simulink library "beamform"  (Simulink 7.0)
libraries: xbsIndex_r4 x65, beamform x13
settings Model: Creator=mdexter  LastModifiedBy=mdexter

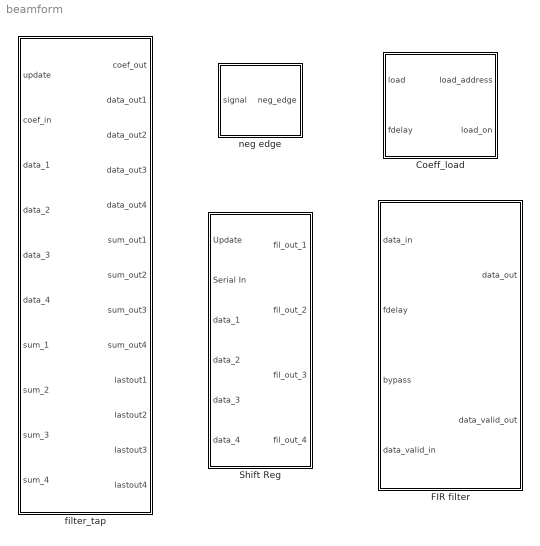
== system beamform ==
  Coeff_load : Subsystem  mask{nfilters=10, ntaps=20}
      mask prompts: nfilters "Number of FD filters"; ntaps "Number of Taps per filter"
      mask init:
      | coef_load;
  FIR filter : Subsystem
  Shift Reg : Subsystem  mask{n=10, bin_point=6}
      mask prompts: n "No of taps"; bin_point "Binary Point"
      mask init:
      | shift_reg;
  filter_tap : Subsystem  mask{n_bits=8, bnpnt=6, mux_latency=0, add_latency=2, mult_latency=3, qn_bits=18, qbnpnt=16}
      mask prompts: n_bits "Coefficient bit width"; bnpnt "Coeff & Data Binary Point"; mux_latency "Multiplexer Latency"; add_latency "Add Latency"; mult_latency "Multiplier Latency"; qn_bits "Quiscent Bitwdith"; qbnpnt "Quiscent Binary Point"
  neg edge : Subsystem  mask{add_latency=1}

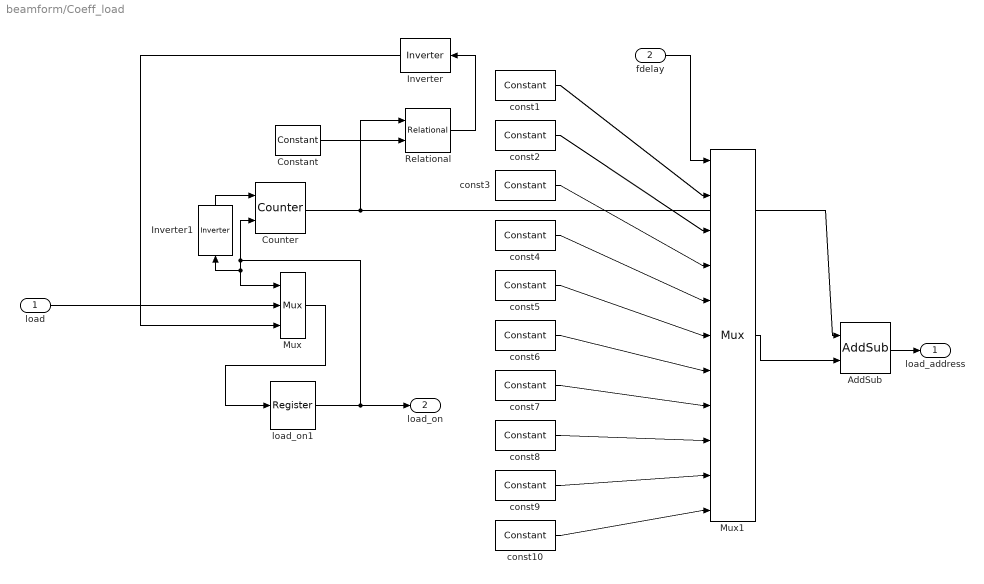
== system beamform/Coeff_load ==
  load : Inport  OutDataType=sfix(16)  OutScaling=2^0
  fdelay : Inport  Port=2  OutDataType=sfix(16)  OutScaling=2^0
  AddSub : xbsIndex_r4/AddSub  mode=Addition  use_carryin=off  use_carryout=off  en=off  latency=1  precision=User Defined  arith_type=Unsigned  n_bits=8  bin_pt=0  quantization=Truncate  overflow=Wrap  dbl_ovrd=off  use_behavioral_HDL=on  pipelined=off  use_rpm=on  hw_selection=Fabric  block_type=addsub
      settings: xl_area=[0, 0, 0, 0, 0, 0, 0]  block_version=10.1.3
  Constant : xbsIndex_r4/Constant  arith_type=Unsigned  const=19  n_bits=5  bin_pt=0  explicit_period=on  period=1  equ=P=C  opselect=C  inp2=PCIN>>17  opr=+  inp1=P  carry=CIN  dbl_ovrd=off  block_type=constant
  Counter : xbsIndex_r4/Counter  cnt_type=Count Limited  cnt_to=19  operation=Up  start_count=0  cnt_by_val=1  arith_type=Unsigned  n_bits=5  bin_pt=0  load_pin=off  rst=on  en=on  explicit_period=off  period=1  dbl_ovrd=off  use_behavioral_HDL=off  use_rpm=on  implementation=Fabric  block_type=counter
      settings: xl_area=[0, 0, 0, 0, 0, 0, 0]
  Inverter : xbsIndex_r4/Inverter  Orientation=left  en=off  latency=0  dbl_ovrd=off  block_type=inv
      settings: xl_area=[0, 0, 0, 0, 0, 0, 0]
  Inverter1 : xbsIndex_r4/Inverter  Orientation=up  en=off  latency=0  dbl_ovrd=off  block_type=inv
      settings: xl_area=[0, 0, 0, 0, 0, 0, 0]
  Mux : xbsIndex_r4/Mux  inputs=2  en=off  latency=0  precision=Full  arith_type="Signed  (2's comp)"  n_bits=8  bin_pt=2  quantization=Truncate  overflow=Wrap  dbl_ovrd=off  block_type=mux
      settings: xl_area=[0, 0, 0, 0, 0, 0, 0]
  Mux1 : xbsIndex_r4/Mux  inputs=10  en=off  latency=1  precision=Full  arith_type="Signed  (2's comp)"  n_bits=8  bin_pt=2  quantization=Truncate  overflow=Wrap  dbl_ovrd=off  block_type=mux
      settings: xl_area=[0, 0, 0, 0, 0, 0, 0]
  Relational : xbsIndex_r4/Relational  mode=a>=b  en=off  latency=1  dbl_ovrd=off  block_type=relational
      settings: xl_area=[0, 0, 0, 0, 0, 0, 0]  block_version=10.1.3
  const1 : xbsIndex_r4/Constant  arith_type=Unsigned  const=0  n_bits=8  bin_pt=0  explicit_period=off  period=1  equ=P=C  opselect=C  inp2=PCIN>>17  opr=+  inp1=P  carry=CIN  dbl_ovrd=off  block_type=constant
  const10 : xbsIndex_r4/Constant  arith_type=Unsigned  const=180  n_bits=8  bin_pt=0  explicit_period=off  period=1  equ=P=C  opselect=C  inp2=PCIN>>17  opr=+  inp1=P  carry=CIN  dbl_ovrd=off  block_type=constant
  const2 : xbsIndex_r4/Constant  arith_type=Unsigned  const=20  n_bits=8  bin_pt=0  explicit_period=off  period=1  equ=P=C  opselect=C  inp2=PCIN>>17  opr=+  inp1=P  carry=CIN  dbl_ovrd=off  block_type=constant
  const3 : xbsIndex_r4/Constant  arith_type=Unsigned  const=40  n_bits=8  bin_pt=0  explicit_period=off  period=1  equ=P=C  opselect=C  inp2=PCIN>>17  opr=+  inp1=P  carry=CIN  dbl_ovrd=off  block_type=constant
  const4 : xbsIndex_r4/Constant  arith_type=Unsigned  const=60  n_bits=8  bin_pt=0  explicit_period=off  period=1  equ=P=C  opselect=C  inp2=PCIN>>17  opr=+  inp1=P  carry=CIN  dbl_ovrd=off  block_type=constant
  const5 : xbsIndex_r4/Constant  arith_type=Unsigned  const=80  n_bits=8  bin_pt=0  explicit_period=off  period=1  equ=P=C  opselect=C  inp2=PCIN>>17  opr=+  inp1=P  carry=CIN  dbl_ovrd=off  block_type=constant
  const6 : xbsIndex_r4/Constant  arith_type=Unsigned  const=100  n_bits=8  bin_pt=0  explicit_period=off  period=1  equ=P=C  opselect=C  inp2=PCIN>>17  opr=+  inp1=P  carry=CIN  dbl_ovrd=off  block_type=constant
  const7 : xbsIndex_r4/Constant  arith_type=Unsigned  const=120  n_bits=8  bin_pt=0  explicit_period=off  period=1  equ=P=C  opselect=C  inp2=PCIN>>17  opr=+  inp1=P  carry=CIN  dbl_ovrd=off  block_type=constant
  const8 : xbsIndex_r4/Constant  arith_type=Unsigned  const=140  n_bits=8  bin_pt=0  explicit_period=off  period=1  equ=P=C  opselect=C  inp2=PCIN>>17  opr=+  inp1=P  carry=CIN  dbl_ovrd=off  block_type=constant
  const9 : xbsIndex_r4/Constant  arith_type=Unsigned  const=160  n_bits=8  bin_pt=0  explicit_period=off  period=1  equ=P=C  opselect=C  inp2=PCIN>>17  opr=+  inp1=P  carry=CIN  dbl_ovrd=off  block_type=constant
  load_on1 : xbsIndex_r4/Register  init=0  rst=off  en=off  dbl_ovrd=off  block_type=register
      settings: xl_area=[0, 0, 0, 0, 0, 0, 0]
  load_address : Outport  OutDataType=sfix(16)  OutScaling=2^0
  load_on : Outport  Port=2  OutDataType=sfix(16)  OutScaling=2^0
  wires:
  const10/1 -> Mux1/11
  const9/1 -> Mux1/10
  const8/1 -> Mux1/9
  const7/1 -> Mux1/8
  const6/1 -> Mux1/7
  const5/1 -> Mux1/6
  const4/1 -> Mux1/5
  const3/1 -> Mux1/4
  const2/1 -> Mux1/3
  const1/1 -> Mux1/2
  AddSub/1 -> load_address/1
  Mux1/1 -> AddSub/2
  fdelay/1 -> Mux1/1
  Inverter1/1 -> Counter/1
  load/1 -> Mux/2
  Mux/1 -> load_on1/1
  Inverter/1 -> Mux/3
  load_on1/1 -> load_on/1, Inverter1/1, Mux/1, Counter/2
  Relational/1 -> Inverter/1
  Constant/1 -> Relational/2
  Counter/1 -> AddSub/1, Relational/1

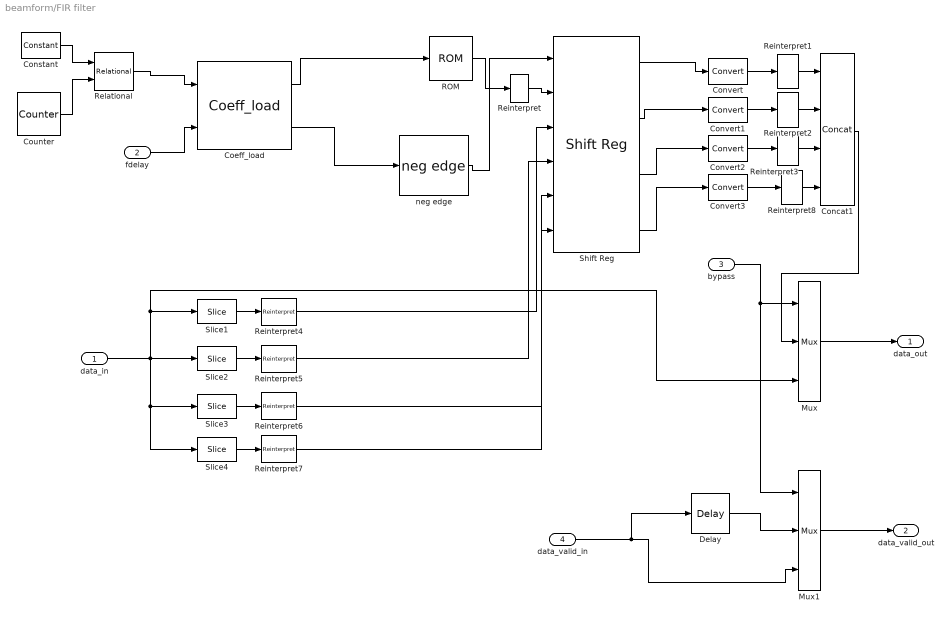
== system beamform/FIR filter ==
  data_in : Inport  OutDataType=sfix(16)  OutScaling=2^0
  fdelay : Inport  Port=2  OutDataType=sfix(16)  OutScaling=2^0
  bypass : Inport  Port=3  OutDataType=sfix(16)  OutScaling=2^0
  data_valid_in : Inport  Port=4  OutDataType=sfix(16)  OutScaling=2^0
  Coeff_load : beamform/Coeff_load  SystemSampleTime=-1  nfilters=10  ntaps=10
  Concat1 : xbsIndex_r4/Concat  num_inputs=4  dbl_ovrd=off  block_type=concat
      settings: block_version=10.1.3
  Constant : xbsIndex_r4/Constant  arith_type=Unsigned  const=0  n_bits=11  bin_pt=0  explicit_period=on  period=1  equ=P=C  opselect=C  inp2=PCIN>>17  opr=+  inp1=P  carry=CIN  dbl_ovrd=off  block_type=constant
  Convert{,1..3} (4 alike) : xbsIndex_r4/Convert  arith_type="Signed  (2's comp)"  n_bits=8  bin_pt=6  quantization=Truncate  overflow=Wrap  latency=0  dbl_ovrd=off  pipeline=off  block_type=convert
      settings: xl_area=[0, 0, 0, 0, 0, 0, 0]  block_version=10.1.3
  Counter : xbsIndex_r4/Counter  cnt_type=Free Running  cnt_to=Inf  operation=Up  start_count=0  cnt_by_val=1  arith_type=Unsigned  n_bits=11  bin_pt=0  load_pin=off  rst=off  en=off  explicit_period=off  period=1  dbl_ovrd=off  use_behavioral_HDL=off  use_rpm=on  implementation=Fabric  block_type=counter
      settings: xl_area=[0, 0, 0, 0, 0, 0, 0]
  Delay : xbsIndex_r4/Delay  en=off  latency=10*6  dbl_ovrd=off  reg_retiming=off  block_type=delay
      settings: xl_area=[0, 0, 0, 0, 0, 0, 0]
  Mux : xbsIndex_r4/Mux  inputs=2  en=off  latency=1  precision=Full  arith_type="Signed  (2's comp)"  n_bits=8  bin_pt=2  quantization=Truncate  overflow=Wrap  dbl_ovrd=off  block_type=mux
      settings: xl_area=[0, 0, 0, 0, 0, 0, 0]
  Mux1 : xbsIndex_r4/Mux  inputs=2  en=off  latency=1  precision=Full  arith_type="Signed  (2's comp)"  n_bits=8  bin_pt=2  quantization=Truncate  overflow=Wrap  dbl_ovrd=off  block_type=mux
      settings: xl_area=[0, 0, 0, 0, 0, 0, 0]
  ROM : xbsIndex_r4/ROM  depth=100  initVector=A  distributed_mem=Block RAM  rst=off  init_reg=0  en=off  latency=1  arith_type="Signed  (2's comp)"  n_bits=18  bin_pt=16  dbl_ovrd=off  optimize=Area  use_rpm=off  block_type=sprom
      settings: xl_area=[0, 0, 0, 0, 0, 0, 0]  block_version=10.1.3
  Reinterpret : xbsIndex_r4/Reinterpret  force_arith_type=on  arith_type="Signed  (2's comp)"  force_bin_pt=on  bin_pt=16  block_type=reinterpret
      settings: infoedit="Changes signal type without altering the binary representation.   You can changed the signal between signed and unsigned, and relocate the binary point.<P><P>Hardware notes: In hardware this block costs nothing.<P><P>Example:  Suppose the input is 6 bits wide, signed, with 2 fractional bits, and the output is forced to unsigned with 0 fractional bits.  Then an input of -2.0 (1110.00 in binary 2's complement) becomes an output of 56 (111000 in binary)."  block_version=10.1.3
  Reinterpret{1..3,8} (4 alike) : xbsIndex_r4/Reinterpret  force_arith_type=on  arith_type=Unsigned  force_bin_pt=on  bin_pt=0  block_type=reinterpret
      settings: infoedit="Changes signal type without altering the binary representation.   You can changed the signal between signed and unsigned, and relocate the binary point.<P><P>Hardware notes: In hardware this block costs nothing.<P><P>Example:  Suppose the input is 6 bits wide, signed, with 2 fractional bits, and the output is forced to unsigned with 0 fractional bits.  Then an input of -2.0 (1110.00 in binary 2's complement) becomes an output of 56 (111000 in binary)."  block_version=10.1.3
  Reinterpret{4..7} (4 alike) : xbsIndex_r4/Reinterpret  force_arith_type=on  arith_type="Signed  (2's comp)"  force_bin_pt=on  bin_pt=6  block_type=reinterpret
      settings: infoedit="Changes signal type without altering the binary representation.   You can changed the signal between signed and unsigned, and relocate the binary point.<P><P>Hardware notes: In hardware this block costs nothing.<P><P>Example:  Suppose the input is 6 bits wide, signed, with 2 fractional bits, and the output is forced to unsigned with 0 fractional bits.  Then an input of -2.0 (1110.00 in binary 2's complement) becomes an output of 56 (111000 in binary)."  block_version=10.1.3
  Relational : xbsIndex_r4/Relational  mode=a=b  en=off  latency=1  dbl_ovrd=off  block_type=relational
      settings: xl_area=[0, 0, 0, 0, 0, 0, 0]  block_version=10.1.3
  Shift Reg : beamform/Shift Reg  SystemSampleTime=-1  n=10  bin_point=6
  Slice1 : xbsIndex_r4/Slice  nbits=8  boolean_output=off  mode=Two Bit Locations  bit1=31  base1=LSB of Input  bit0=24  base0=LSB of Input  dbl_ovrd=off  block_type=slice
      settings: infoedit="Extracts a given range of bits from each input sample and presents it at the output.  The output type is ordinarily unsigned with binary point at zero, but can be Boolean when the slice is one bit wide.<P><P>Hardware notes: In hardware this block costs nothing."  block_version=10.1.3
  Slice2 : xbsIndex_r4/Slice  nbits=8  boolean_output=off  mode=Two Bit Locations  bit1=23  base1=LSB of Input  bit0=16  base0=LSB of Input  dbl_ovrd=off  block_type=slice
      settings: infoedit="Extracts a given range of bits from each input sample and presents it at the output.  The output type is ordinarily unsigned with binary point at zero, but can be Boolean when the slice is one bit wide.<P><P>Hardware notes: In hardware this block costs nothing."  block_version=10.1.3
  Slice3 : xbsIndex_r4/Slice  nbits=8  boolean_output=off  mode=Two Bit Locations  bit1=15  base1=LSB of Input  bit0=8  base0=LSB of Input  dbl_ovrd=off  block_type=slice
      settings: infoedit="Extracts a given range of bits from each input sample and presents it at the output.  The output type is ordinarily unsigned with binary point at zero, but can be Boolean when the slice is one bit wide.<P><P>Hardware notes: In hardware this block costs nothing."  block_version=10.1.3
  Slice4 : xbsIndex_r4/Slice  nbits=8  boolean_output=off  mode=Two Bit Locations  bit1=7  base1=LSB of Input  bit0=0  base0=LSB of Input  dbl_ovrd=off  block_type=slice
      settings: infoedit="Extracts a given range of bits from each input sample and presents it at the output.  The output type is ordinarily unsigned with binary point at zero, but can be Boolean when the slice is one bit wide.<P><P>Hardware notes: In hardware this block costs nothing."  block_version=10.1.3
  neg edge : beamform/neg edge  SystemSampleTime=-1  add_latency=1
  data_out : Outport  OutDataType=sfix(16)  OutScaling=2^0
  data_valid_out : Outport  Port=2  OutDataType=sfix(16)  OutScaling=2^0
  wires:
  Reinterpret/1 -> Shift Reg/2
  neg edge/1 -> Shift Reg/1
  Relational/1 -> Coeff_load/1
  Coeff_load/1 -> ROM/1
  ROM/1 -> Reinterpret/1
  Coeff_load/2 -> neg edge/1
  fdelay/1 -> Coeff_load/2
  Slice1/1 -> Reinterpret4/1
  Slice2/1 -> Reinterpret5/1
  Slice3/1 -> Reinterpret6/1
  Slice4/1 -> Reinterpret7/1
  data_in/1 -> Slice2/1, Slice3/1, Slice4/1, Slice1/1, Mux/3
  Reinterpret4/1 -> Shift Reg/3
  Reinterpret5/1 -> Shift Reg/4
  Reinterpret6/1 -> Shift Reg/5
  Reinterpret7/1 -> Shift Reg/6
  Shift Reg/1 -> Convert/1
  Shift Reg/2 -> Convert1/1
  Shift Reg/3 -> Convert2/1
  Shift Reg/4 -> Convert3/1
  Convert/1 -> Reinterpret1/1
  Convert1/1 -> Reinterpret2/1
  Convert2/1 -> Reinterpret3/1
  Convert3/1 -> Reinterpret8/1
  Mux/1 -> data_out/1
  bypass/1 -> Mux/1, Mux1/1
  Concat1/1 -> Mux/2
  Reinterpret1/1 -> Concat1/1
  Reinterpret2/1 -> Concat1/2
  Reinterpret3/1 -> Concat1/3
  Reinterpret8/1 -> Concat1/4
  data_valid_in/1 -> Mux1/3, Delay/1
  Delay/1 -> Mux1/2
  Mux1/1 -> data_valid_out/1
  Constant/1 -> Relational/1
  Counter/1 -> Relational/2

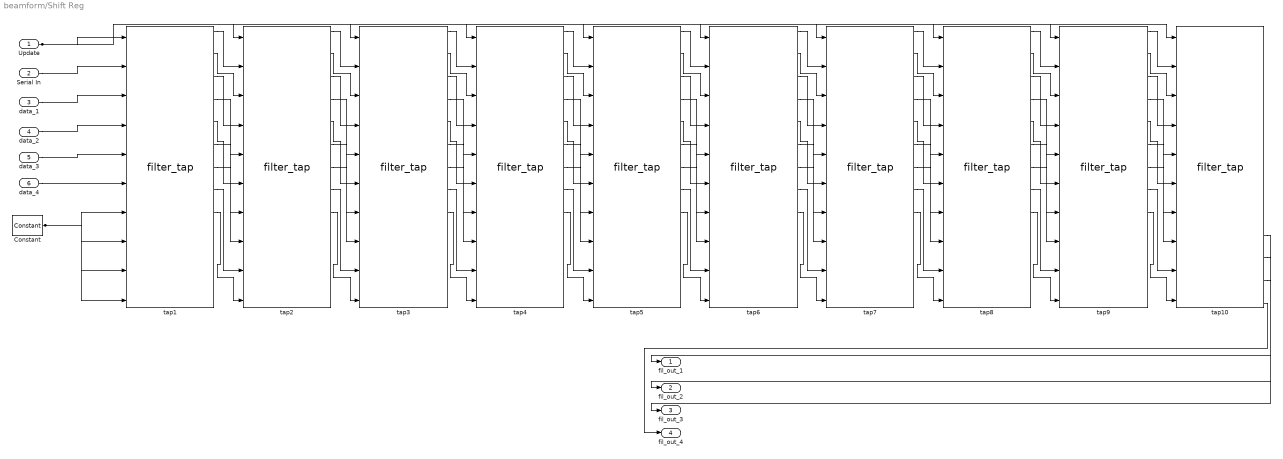
== system beamform/Shift Reg ==
  Update : Inport  OutDataType=sfix(16)  OutScaling=2^0
  Serial In : Inport  Port=2  OutDataType=sfix(16)  OutScaling=2^0
  data_1 : Inport  Port=3  OutDataType=sfix(16)  OutScaling=2^0
  data_2 : Inport  Port=4  OutDataType=sfix(16)  OutScaling=2^0
  data_3 : Inport  Port=5  OutDataType=sfix(16)  OutScaling=2^0
  data_4 : Inport  Port=6  OutDataType=sfix(16)  OutScaling=2^0
  Constant : xbsIndex_r4/Constant  arith_type=Signed (2's comp)  const=0  n_bits=18  bin_pt=6  explicit_period=on  period=1  equ=P=C  opselect=C  inp2=PCIN>>17  opr=+  inp1=P  carry=CIN  dbl_ovrd=off  block_type=constant
  tap{1..10} (10 alike) : beamform/filter_tap  SystemSampleTime=-1  n_bits=8  bnpnt=6  mux_latency=0  add_latency=2  mult_latency=3  qn_bits=18  qbnpnt=16
  fil_out_1 : Outport  OutDataType=sfix(16)  OutScaling=2^0
  fil_out_2 : Outport  Port=2  OutDataType=sfix(16)  OutScaling=2^0
  fil_out_3 : Outport  Port=3  OutDataType=sfix(16)  OutScaling=2^0
  fil_out_4 : Outport  Port=4  OutDataType=sfix(16)  OutScaling=2^0
  wires:
  Update/1 -> tap1/1, tap2/1, tap3/1, tap4/1, tap5/1, tap6/1, tap7/1, tap8/1, tap9/1, tap10/1
  Serial In/1 -> tap1/2
  data_1/1 -> tap1/3
  data_2/1 -> tap1/4
  data_3/1 -> tap1/5
  data_4/1 -> tap1/6
  Constant/1 -> tap1/7, tap1/8, tap1/9, tap1/10
  tap1/1 -> tap2/2
  tap1/2 -> tap2/3
  tap1/3 -> tap2/4
  tap1/4 -> tap2/5
  tap1/5 -> tap2/6
  tap1/6 -> tap2/7
  tap1/7 -> tap2/8
  tap1/8 -> tap2/9
  tap1/9 -> tap2/10
  tap2/1 -> tap3/2
  tap2/2 -> tap3/3
  tap2/3 -> tap3/4
  tap2/4 -> tap3/5
  tap2/5 -> tap3/6
  tap2/6 -> tap3/7
  tap2/7 -> tap3/8
  tap2/8 -> tap3/9
  tap2/9 -> tap3/10
  tap3/1 -> tap4/2
  tap3/2 -> tap4/3
  tap3/3 -> tap4/4
  tap3/4 -> tap4/5
  tap3/5 -> tap4/6
  tap3/6 -> tap4/7
  tap3/7 -> tap4/8
  tap3/8 -> tap4/9
  tap3/9 -> tap4/10
  tap4/1 -> tap5/2
  tap4/2 -> tap5/3
  tap4/3 -> tap5/4
  tap4/4 -> tap5/5
  tap4/5 -> tap5/6
  tap4/6 -> tap5/7
  tap4/7 -> tap5/8
  tap4/8 -> tap5/9
  tap4/9 -> tap5/10
  tap5/1 -> tap6/2
  tap5/2 -> tap6/3
  tap5/3 -> tap6/4
  tap5/4 -> tap6/5
  tap5/5 -> tap6/6
  tap5/6 -> tap6/7
  tap5/7 -> tap6/8
  tap5/8 -> tap6/9
  tap5/9 -> tap6/10
  tap6/1 -> tap7/2
  tap6/2 -> tap7/3
  tap6/3 -> tap7/4
  tap6/4 -> tap7/5
  tap6/5 -> tap7/6
  tap6/6 -> tap7/7
  tap6/7 -> tap7/8
  tap6/8 -> tap7/9
  tap6/9 -> tap7/10
  tap7/1 -> tap8/2
  tap7/2 -> tap8/3
  tap7/3 -> tap8/4
  tap7/4 -> tap8/5
  tap7/5 -> tap8/6
  tap7/6 -> tap8/7
  tap7/7 -> tap8/8
  tap7/8 -> tap8/9
  tap7/9 -> tap8/10
  tap8/1 -> tap9/2
  tap8/2 -> tap9/3
  tap8/3 -> tap9/4
  tap8/4 -> tap9/5
  tap8/5 -> tap9/6
  tap8/6 -> tap9/7
  tap8/7 -> tap9/8
  tap8/8 -> tap9/9
  tap8/9 -> tap9/10
  tap9/1 -> tap10/2
  tap9/2 -> tap10/3
  tap9/3 -> tap10/4
  tap9/4 -> tap10/5
  tap9/5 -> tap10/6
  tap9/6 -> tap10/7
  tap9/7 -> tap10/8
  tap9/8 -> tap10/9
  tap9/9 -> tap10/10
  tap10/10 -> fil_out_1/1
  tap10/11 -> fil_out_2/1
  tap10/12 -> fil_out_3/1
  tap10/13 -> fil_out_4/1

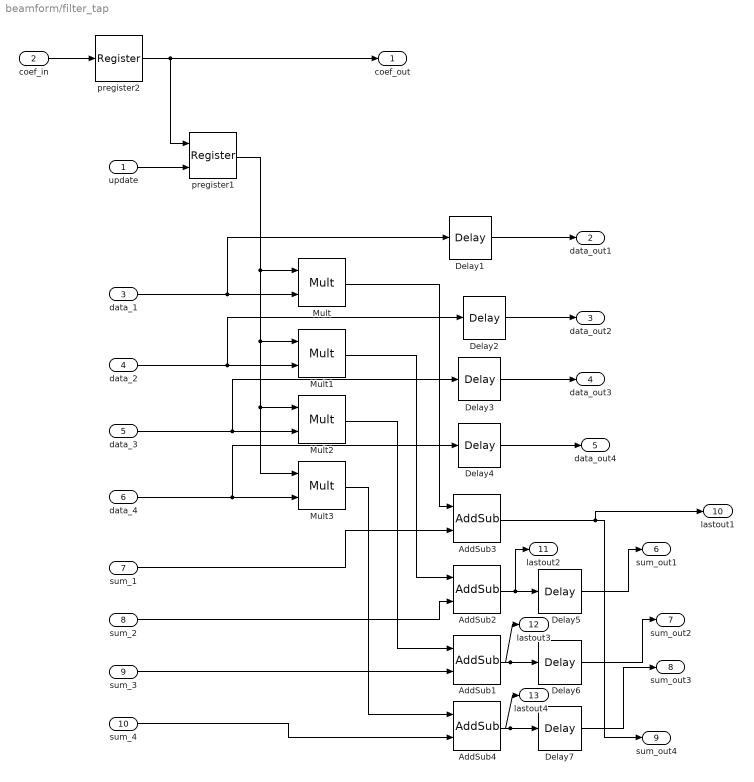
== system beamform/filter_tap ==
  update : Inport  OutDataType=sfix(16)  OutScaling=2^0
  coef_in : Inport  Port=2  OutDataType=sfix(16)  OutScaling=2^0
  data_1 : Inport  Port=3  OutDataType=sfix(16)  OutScaling=2^0
  data_2 : Inport  Port=4  OutDataType=sfix(16)  OutScaling=2^0
  data_3 : Inport  Port=5  OutDataType=sfix(16)  OutScaling=2^0
  data_4 : Inport  Port=6  OutDataType=sfix(16)  OutScaling=2^0
  sum_1 : Inport  Port=7  OutDataType=sfix(16)  OutScaling=2^0
  sum_2 : Inport  Port=8  OutDataType=sfix(16)  OutScaling=2^0
  sum_3 : Inport  Port=9  OutDataType=sfix(16)  OutScaling=2^0
  sum_4 : Inport  Port=10  OutDataType=sfix(16)  OutScaling=2^0
  AddSub{1..4} (4 alike) : xbsIndex_r4/AddSub  mode=Addition  use_carryin=off  use_carryout=off  en=off  latency=add_latency  precision=User Defined  arith_type="Signed  (2's comp)"  n_bits=qn_bits  bin_pt=qbnpnt  quantization=Truncate  overflow=Wrap  dbl_ovrd=off  use_behavioral_HDL=on  pipelined=off  use_rpm=on  hw_selection=Fabric  block_type=addsub
      settings: xl_area=[0, 0, 0, 0, 0, 0, 0]  block_version=10.1.3
  Delay{1..4} (4 alike) : xbsIndex_r4/Delay  en=off  latency=add_latency+1  dbl_ovrd=off  reg_retiming=on  block_type=delay
      settings: xl_area=[0, 0, 0, 0, 0, 0, 0]
  Delay5 : xbsIndex_r4/Delay  en=off  latency=1  dbl_ovrd=off  reg_retiming=on  block_type=delay
      settings: xl_area=[0, 0, 0, 0, 0, 0, 0]
  Delay6 : xbsIndex_r4/Delay  en=off  latency=1  dbl_ovrd=off  reg_retiming=on  block_type=delay
      settings: xl_area=[0, 0, 0, 0, 0, 0, 0]
  Delay7 : xbsIndex_r4/Delay  en=off  latency=1  dbl_ovrd=off  reg_retiming=on  block_type=delay
      settings: xl_area=[0, 0, 0, 0, 0, 0, 0]
  Mult{,1..3} (4 alike) : xbsIndex_r4/Mult  precision=User Defined  arith_type="Signed  (2's comp)"  n_bits=n_bits  bin_pt=bnpnt  quantization=Truncate  overflow=Wrap  en=off  latency=mult_latency  dbl_ovrd=off  use_behavioral_HDL=off  use_embedded=on  opt=Speed  optimum_pipeline=off  pipeline=on  use_rpm=on  placement_style=Rectangular shape  block_type=mult
      settings: infoedit=Hardware notes: To use the internal pipeline stage of the dedicated multiplier you must select 'Pipeline for maximum performance'.  xl_area=[0, 0, 0, 0, 0, 0, 0]  block_version=10.1.3
  pregister1 : xbsIndex_r4/Register  init=0  rst=off  en=on  dbl_ovrd=off  block_type=register
      settings: xl_area=[0, 0, 0, 0, 0, 0, 0]
  pregister2 : xbsIndex_r4/Register  init=0  rst=off  en=off  dbl_ovrd=off  block_type=register
      settings: xl_area=[0, 0, 0, 0, 0, 0, 0]
  coef_out : Outport  OutDataType=sfix(16)  OutScaling=2^0
  data_out1 : Outport  Port=2  OutDataType=sfix(16)  OutScaling=2^0
  data_out2 : Outport  Port=3  OutDataType=sfix(16)  OutScaling=2^0
  data_out3 : Outport  Port=4  OutDataType=sfix(16)  OutScaling=2^0
  data_out4 : Outport  Port=5  OutDataType=sfix(16)  OutScaling=2^0
  sum_out1 : Outport  Port=6  OutDataType=sfix(16)  OutScaling=2^0
  sum_out2 : Outport  Port=7  OutDataType=sfix(16)  OutScaling=2^0
  sum_out3 : Outport  Port=8  OutDataType=sfix(16)  OutScaling=2^0
  sum_out4 : Outport  Port=9  OutDataType=sfix(16)  OutScaling=2^0
  lastout1 : Outport  Port=10  OutDataType=sfix(16)  OutScaling=2^0
  lastout2 : Outport  Port=11  OutDataType=sfix(16)  OutScaling=2^0
  lastout3 : Outport  Port=12  OutDataType=sfix(16)  OutScaling=2^0
  lastout4 : Outport  Port=13  OutDataType=sfix(16)  OutScaling=2^0
  wires:
  update/1 -> pregister1/2
  Delay7/1 -> sum_out3/1
  Delay6/1 -> sum_out2/1
  Delay5/1 -> sum_out1/1
  AddSub4/1 -> lastout4/1, Delay7/1
  AddSub1/1 -> lastout3/1, Delay6/1
  AddSub2/1 -> lastout2/1, Delay5/1
  AddSub3/1 -> sum_out4/1, lastout1/1
  sum_4/1 -> AddSub4/2
  sum_3/1 -> AddSub1/2
  sum_2/1 -> AddSub2/2
  sum_1/1 -> AddSub3/2
  Delay4/1 -> data_out4/1
  Delay3/1 -> data_out3/1
  Delay2/1 -> data_out2/1
  Delay1/1 -> data_out1/1
  Mult3/1 -> AddSub4/1
  Mult/1 -> AddSub3/1
  Mult1/1 -> AddSub2/1
  Mult2/1 -> AddSub1/1
  data_4/1 -> Delay4/1, Mult3/2
  data_3/1 -> Delay3/1, Mult2/2
  data_2/1 -> Delay2/1, Mult1/2
  data_1/1 -> Delay1/1, Mult/2
  pregister2/1 -> pregister1/1, coef_out/1
  coef_in/1 -> pregister2/1
  pregister1/1 -> Mult1/1, Mult3/1, Mult2/1, Mult/1

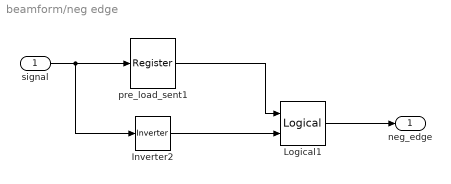
== system beamform/neg edge ==
  signal : Inport  OutDataType=sfix(16)  OutScaling=2^0
  Inverter2 : xbsIndex_r4/Inverter  en=off  latency=0  dbl_ovrd=off  block_type=inv
      settings: xl_area=[0, 0, 0, 0, 0, 0, 0]
  Logical1 : xbsIndex_r4/Logical  logical_function=AND  inputs=2  en=off  latency=add_latency  precision=Full  arith_type=Unsigned  n_bits=8  bin_pt=2  align_bp=on  dbl_ovrd=off  block_type=logical
      settings: xl_area=[0, 0, 0, 0, 0, 0, 0]
  pre_load_sent1 : xbsIndex_r4/Register  init=0  rst=off  en=off  dbl_ovrd=off  block_type=register
      settings: xl_area=[0, 0, 0, 0, 0, 0, 0]
  neg_edge : Outport  OutDataType=sfix(16)  OutScaling=2^0
  wires:
  Inverter2/1 -> Logical1/2
  signal/1 -> Inverter2/1, pre_load_sent1/1
  pre_load_sent1/1 -> Logical1/1
  Logical1/1 -> neg_edge/1
